simulink model "chap3_1sim"  (R2016b)
settings: Solver=ode45  StartTime=0.0  StopTime=RunTime  FixedStep=0.01  RelTol=1e-3  EnableMultiTasking=on
settings Model: Creator=Masoud  LastModifiedBy=Hafez
settings DataIOCC: LimitDataPoints=on  SaveFormat=Array
settings OptimizationCC: LifeSpan=inf
settings DebuggingCC: SFUnexpectedBacktrackingDiag=warning  SFNoUnconditionalDefaultTransitionDiag=warning  SFExecutionAtInitializationDiag=none
settings HardwareCC: ProdBitPerPointer=32  ProdBitPerSizeT=32  ProdBitPerPtrDiffT=32  ProdLargestAtomicFloat=None  ProdIntDivRoundTo=Undefined  ProdEndianess=Unspecified  ProdWordSize=32  ProdHWDeviceType=32-bit Generic
settings ModelReferenceCC: PropagateSignalLabelsOutOfModel=off
settings GRTTargetCC: TargetLangStandard=C89/C90 (ANSI)  GeneratePreprocessorConditionals=Disable all
settings ConfigComp: CovMetricSettings=dw  CovHtmlReporting=on  CovSaveCumulativeToWorkspaceVar=on  CovSaveSingleToWorkspaceVar=on  CovExternalEMLEnable=off

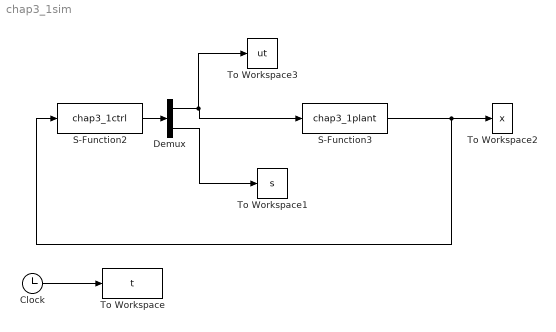
== system chap3_1sim ==
  Clock : Clock
  Demux : Demux  Outputs=2
  S-Function2 : S-Function  FunctionName=chap3_1ctrl  SFunctionModules='chap3_1ctrl'  SFunctionDeploymentMode=off  EnableBusSupport=off
  S-Function3 : S-Function  FunctionName=chap3_1plant  SFunctionModules='chap3_1plant'  SFunctionDeploymentMode=off  EnableBusSupport=off
  To Workspace : ToWorkspace  VariableName=t  SampleTime=-1
  To Workspace1 : ToWorkspace  VariableName=s  SampleTime=-1
  To Workspace2 : ToWorkspace  VariableName=x  SampleTime=-1
  To Workspace3 : ToWorkspace  VariableName=ut  SampleTime=-1
  wires:
  Clock/1 -> To Workspace/1
  S-Function3/1 -> S-Function2/1, To Workspace2/1
  S-Function2/1 -> Demux/1
  Demux/1 -> To Workspace3/1, S-Function3/1
  Demux/2 -> To Workspace1/1
